simulink model "practice2"  (R2020b)
settings: Solver=FixedStepDiscrete  StartTime=0.0  StopTime=10.0  FixedStep=0.1  RelTol=1e-3  EnableMultiTasking=on
settings Model: Creator=yuto  LastModifiedBy=yuto
settings SolverCC: AutoInsertRateTranBlk=on
settings DataIOCC: LimitDataPoints=on
settings OptimizationCC: LifeSpan=inf
settings DebuggingCC: AllowSymbolicDim=off  SFUnexpectedBacktrackingDiag=warning  SFNoUnconditionalDefaultTransitionDiag=warning  SFExecutionAtInitializationDiag=none  ArithmeticOperatorsInVariantConditions=warning
settings SFSimCC: SimUseLocalCustomCode=off  CustomCodeUndefinedFunction=UseInterfaceOnly
settings RTWCC: RTWUseLocalCustomCode=off
settings CodeAppCC: StateflowObjectComments=on
settings GRTTargetCC: TargetLangStandard=C89/C90 (ANSI)
settings ConfigComp: CovMetricSettings=dw  CovSaveCumulativeToWorkspaceVar=on  CovSaveSingleToWorkspaceVar=on  CovExternalEMLEnable=off  CovSFcnEnable=off

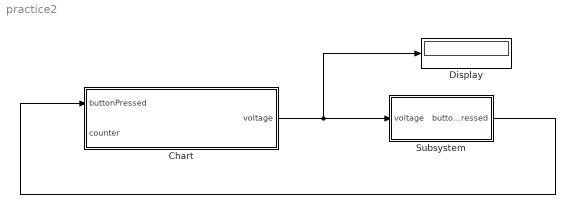
== system practice2 ==
  Chart : Stateflow chart  TreatAsAtomicUnit=on
  Display : Display
  Subsystem : Subsystem
  wires:
  Chart/1(voltage) -> Display/1, Subsystem/1(voltage)
  Subsystem/1(buttonPressed) -> Chart/1(buttonPressed)

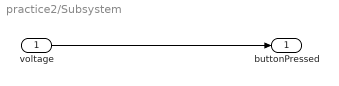
== system practice2/Subsystem ==
  voltage : Inport
  buttonPressed : Outport
  wires:
  voltage/1 -> buttonPressed/1

== stateflow chart practice2/Chart ==
  state turnOn1
    entry:voltage=1;
  state turnOff
    entry:voltage=-1;
    counter = counter + 1
  (default) -> turnOn1
  turnOn1 -> turnOff : [buttonPressed==1]
  turnOff -> turnOn1 : [buttonPressed==0]
  data: voltage output; buttonPressed input; counter input
